simulink model "PDU_Logic_Design"  (R2024b)
settings: Solver=VariableStepAuto  StartTime=0.0  StopTime=10.0  RelTol=1e-3
libraries: spsVoltageMeasurementLib x4, spsCurrentMeasurementLib x3, spsIdealSwitchLib x3, spsControlledVoltageSourceLib x2, spsGroundLib x2, spsSeriesRLCBranchLib x1, sps_lib x1

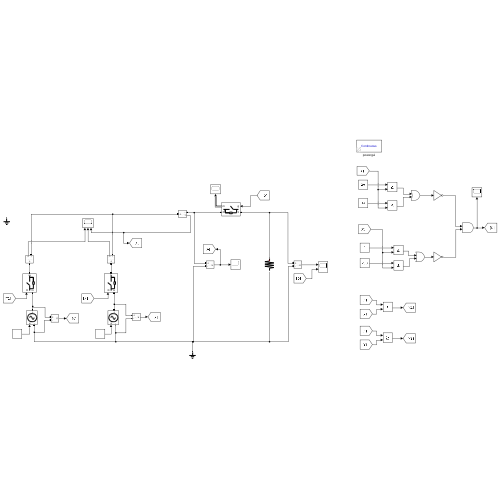
[thumbnail: Simulink's stored preview of the top-level diagram]
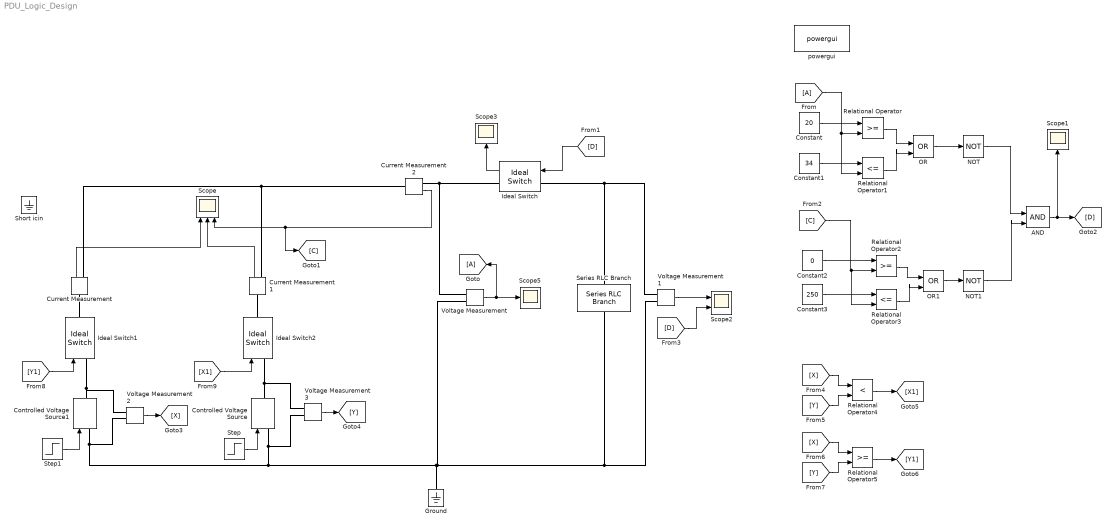
== system PDU_Logic_Design ==
  AND : Logic  IconShape=distinctive  AllPortsSameDT=off  OutDataTypeStr=boolean
  Constant : Constant  Value=20
  Constant1 : Constant  Value=34
  Constant2 : Constant  Value=0
  Constant3 : Constant  Value=250
  Controlled Voltage Source : spsControlledVoltageSourceLib/Controlled Voltage Source  Initialize=on  Source_Type=DC  Amplitude=0  Phase=0  Frequency=0  Measurements=None
  Controlled Voltage Source1 : spsControlledVoltageSourceLib/Controlled Voltage Source  Initialize=on  Source_Type=DC  Amplitude=0  Phase=0  Frequency=0  Measurements=None
  Current Measurement : spsCurrentMeasurementLib/Current Measurement  PhasorSimulation=off  OutputType=Complex  PSBequivalent=0
  Current Measurement1 : spsCurrentMeasurementLib/Current Measurement  PhasorSimulation=off  OutputType=Complex  PSBequivalent=0
  Current Measurement2 : spsCurrentMeasurementLib/Current Measurement  PhasorSimulation=off  OutputType=Complex  PSBequivalent=0
  From : From
  Goto : Goto
  Ground : spsGroundLib/Ground  LConnTagsString=a
  Ideal Switch : spsIdealSwitchLib/Ideal Switch  Ron=0.001  Lon=0  IC=1  Rs=1e5  Cs=inf  Measurements=on
  Ideal Switch1 : spsIdealSwitchLib/Ideal Switch  Ron=0.001  Lon=0  IC=0  Rs=1e5  Cs=inf  Measurements=off
  Ideal Switch2 : spsIdealSwitchLib/Ideal Switch  Ron=0.001  Lon=0  IC=0  Rs=1e5  Cs=inf  Measurements=off
  NOT : Logic  Operator=NOT  IconShape=distinctive  AllPortsSameDT=off  OutDataTypeStr=boolean
  NOT1 : Logic  Operator=NOT  IconShape=distinctive  AllPortsSameDT=off  OutDataTypeStr=boolean
  OR : Logic  Operator=OR  IconShape=distinctive  AllPortsSameDT=off  OutDataTypeStr=boolean
  OR1 : Logic  Operator=OR  IconShape=distinctive  AllPortsSameDT=off  OutDataTypeStr=boolean
  Relational Operator : RelationalOperator  OutDataTypeStr=boolean  RndMeth=Simplest  InputSameDT=off
  Relational Operator1 : RelationalOperator  Operator=<=  OutDataTypeStr=boolean  RndMeth=Simplest  InputSameDT=off
  Relational Operator2 : RelationalOperator  OutDataTypeStr=boolean  RndMeth=Simplest  InputSameDT=off
  Relational Operator3 : RelationalOperator  Operator=<=  OutDataTypeStr=boolean  RndMeth=Simplest  InputSameDT=off
  Relational Operator4 : RelationalOperator  Operator=<  OutDataTypeStr=boolean  RndMeth=Simplest  InputSameDT=off
  Relational Operator5 : RelationalOperator  OutDataTypeStr=boolean  RndMeth=Simplest  InputSameDT=off
  Scope : Scope  NumInputPorts=3
  Scope1 : Scope
  Scope2 : Scope  NumInputPorts=2
  Scope3 : Scope
  Scope5 : Scope
  Series RLC Branch : spsSeriesRLCBranchLib/Series RLC Branch  LConnTagsString=__new0  RConnTagsString=__new0  BranchType=R  Resistance=1  Inductance=1e-3  SetiL0=off  InitialCurrent=0  Capacitance=1e-6  Setx0=off  InitialVoltage=0  Measurements=None
  Short icin : spsGroundLib/Ground  LConnTagsString=a
  Step : Step  Time=4  Before=28  After=10  SampleTime=0
  Step1 : Step  Time=8  Before=26  After=10  SampleTime=0
  Voltage Measurement{,1..3} (4 alike) : spsVoltageMeasurementLib/Voltage Measurement  PhasorSimulation=off  OutputType=Complex  PSBequivalent=0
  powergui : sps_lib/powergui  Priority=1  SimulationMode=Continuous  SampleTime=50e-6  frequency=60  Iterations=50  frequencyindice=0  Pbase=100e6  ErrMax=1e-4  UnitsV=kV  UnitsW=MW  buscounter=0  FunctionMessages=off  echomessages=off  EnableUseOfTLC=off  CurrentSourceSwitches=off  DisableSnubberDevices=off  DisableRonSwitches=off  DisableVfSwitches=off  DisplayEquations=off  AutomaticDiscreteSolvers=off  SolverType=Tustin/Backward Euler (TBE)  Interpol=off  ExternalGateDelay=off  methode=off  Ts=100  x0status=blocks  SPID=on  SwTol=0  HookPort=off  NonlinearTolerance=1e-4  nMaxIteration=100  ContinueOnMaxIteration=off  RestoreLinks=warning  ResistiveCurrentMeasurement=off  Frange=[0:2:500]  Ylog=off  Xlog=on  ShowGrid=off  save=off  variable=ZData  structure=0  ZoomFFT=off  StartTime=0.0  cycles=1  DisplayStyle=1  fundamental=60  FreqAxis=off  MaxFrequency=1000  frequencyindicesteady=1  RmsSteady=1  display=off
  wires:
  Step/1 -> Controlled Voltage Source/1
  Constant/1 -> Relational Operator/1
  Constant1/1 -> Relational Operator1/1
  From/1 -> Relational Operator/2, Relational Operator1/2
  Relational Operator/1 -> OR/1
  Relational Operator1/1 -> OR/2
  OR/1 -> NOT/1
  NOT/1 -> AND/1
  Ideal Switch/1 -> Scope3/1
  Voltage Measurement/1 -> Goto/1, Scope5/1
  Voltage Measurement1/1 -> Scope2/1
  Step1/1 -> Controlled Voltage Source1/1
  Current Measurement/1 -> Scope/1
  Current Measurement1/1 -> Scope/2
  Current Measurement2/1 -> Scope/3, [C]
  [C] -> Relational Operator3/2, Relational Operator2/2
  Constant2/1 -> Relational Operator2/1
  Constant3/1 -> Relational Operator3/1
  Relational Operator2/1 -> OR1/1
  Relational Operator3/1 -> OR1/2
  OR1/1 -> NOT1/1
  NOT1/1 -> AND/2
  AND/1 -> [D], Scope1/1
  [D] -> Ideal Switch/1
  [D] -> Scope2/2
  Voltage Measurement2/1 -> [X]
  Voltage Measurement3/1 -> [Y]
  [X] -> Relational Operator4/1
  [Y] -> Relational Operator4/2
  Relational Operator4/1 -> [X1]
  [X] -> Relational Operator5/1
  Relational Operator5/1 -> [Y1]
  [Y] -> Relational Operator5/2
  [Y1] -> Ideal Switch1/1
  [X1] -> Ideal Switch2/1
  connections:
  Ideal Switch/LConn1 -- Voltage Measurement1/LConn1 -- Series RLC Branch/LConn1
  Series RLC Branch/RConn1 -- Voltage Measurement1/LConn2 -- Voltage Measurement/LConn2 -- Controlled Voltage Source1/LConn1 -- Voltage Measurement2/LConn2 -- Controlled Voltage Source/LConn1 -- Voltage Measurement3/LConn2 -- Ground/LConn1
  Ideal Switch1/LConn1 -- Voltage Measurement2/LConn1 -- Controlled Voltage Source1/RConn1
  Current Measurement2/LConn1 -- Current Measurement/RConn1 -- Current Measurement1/RConn1
  Ideal Switch2/LConn1 -- Voltage Measurement3/LConn1 -- Controlled Voltage Source/RConn1
  Voltage Measurement/LConn1 -- Current Measurement2/RConn1 -- Ideal Switch/RConn1
  Ideal Switch2/RConn1 -- Current Measurement1/LConn1
  Ideal Switch1/RConn1 -- Current Measurement/LConn1
